simulink model "System"  (R2018b)
settings: Solver=FixedStepDiscrete  StartTime=0.0  StopTime=10  RelTol=1e-3
libraries: dspsrcs4 x3
settings Model: Creator=Whtest  LastModifiedBy=Whtest
settings OptimizationCC: DefaultParameterBehavior=Inlined  UseDivisionForNetSlopeComputation=on  UseFloatMulNetSlope=on  InlineInvariantSignals=on  PassReuseOutputArgsAs=Individual arguments  ZeroExternalMemoryAtStartup=off  ZeroInternalMemoryAtStartup=off  NoFixptDivByZeroProtection=on  EfficientFloat2IntCast=on  LifeSpan=1  OptimizeBlockOrder=speed  DifferentSizesBufferReuse=on
settings DebuggingCC: ParameterTunabilityLossMsg=error
settings HardwareCC: ProdBitPerPointer=32  ProdBitPerSizeT=32  ProdBitPerPtrDiffT=32  ProdWordSize=32  ProdLongLongMode=on  ProdHWDeviceType=Intel->x86-32 (Windows32)
settings SFSimCC: MATLABDynamicMemAlloc=off
settings RTWCC: SystemTargetFile=ert.tlc  TemplateMakefile=ert_default_tmf  GenerateReport=on  IncludeHyperlinkInReport=on  LaunchReport=on  GenerateTraceInfo=on  GenerateTraceReport=on  GenerateTraceReportSl=on  GenerateTraceReportSf=on  GenerateTraceReportEml=on  GenerateCodeMetricsReport=on
settings CodeAppCC: ForceParamTrailComments=on  IgnoreCustomStorageClasses=off  OperatorAnnotations=on  SimulinkDataObjDesc=on  SFDataObjDesc=on  CustomSymbolStrGlobalVar=rt$N$M  CustomSymbolStrType=$N$M  CustomSymbolStrFcn=$N$M$F  CustomSymbolStrMacro=$N$M  InsertBlockDesc=on
settings ERTTargetCC: TargetLangStandard=C99 (ISO)  GenerateSampleERTMain=on  IncludeMdlTerminateFcn=off  CombineSignalStateStructs=on  SupportComplex=off  SupportNonInlinedSFcns=on  InlinedParameterPlacement=NonHierarchical  ERTCustomFileTemplate=example_file_process.tlc  ERTFilePackagingFormat=CompactWithDataFile

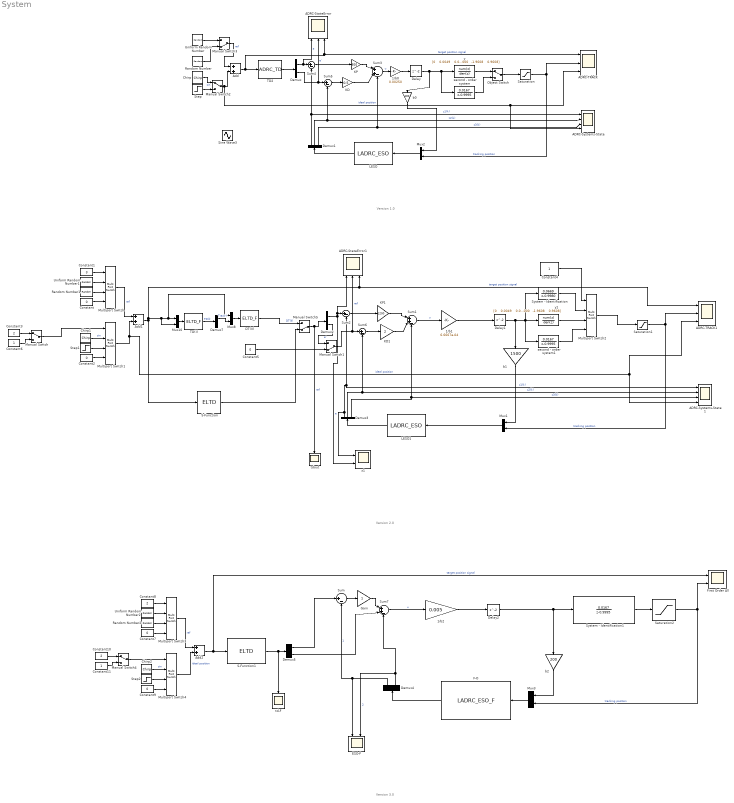
== system System ==
  note: Version 1.0
  note: Version 2.0
  note: Version 3.0
  1/b0 : Gain  Gain=0.00250
  1/b1 : Gain  Gain=6.6667e-04
  1/b2 : Gain  Gain=0.005
  ADRC-StateError : Scope  NumInputPorts=3
  ADRC-StateError1 : Scope  NumInputPorts=3
  "ADRC-Systems-State " : Scope  NumInputPorts=4
  ADRC-Systems-State 1 : Scope  NumInputPorts=4
  ADRC-TRACK : Scope  NumInputPorts=3
  ADRC-TRACK1 : Scope  NumInputPorts=3
  Add : Sum
  Add1 : Sum
  Add2 : Sum
  Chirp : dspsrcs4/Chirp  sweep=Linear  mode=Unidirectional  f0=1  f1=5  t1=5  Tsweep=5  phase=1.5*pi  Ts=0.001  spf=1  datatype=Double  OutputFrames=off
      settings: SourceProductName=DSP System Toolbox
  Chirp1 : dspsrcs4/Chirp  sweep=Linear  mode=Unidirectional  f0=1  f1=5  t1=5  Tsweep=5  phase=1.5*pi  Ts=0.001  spf=1  datatype=Double  OutputFrames=off
      settings: SourceProductName=DSP System Toolbox
  Chirp2 : dspsrcs4/Chirp  sweep=Linear  mode=Unidirectional  f0=1  f1=5  t1=5  Tsweep=5  phase=1.5*pi  Ts=0.001  spf=1  datatype=Double  OutputFrames=off
      settings: SourceProductName=DSP System Toolbox
  Constant{,2,5,7,9} (5 alike) : Constant  Value=0
  Constant1 : Constant  Value=3
  Constant10 : Constant  Value=2
  Constant11 : Constant
  Constant3 : Constant  Value=2
  Constant4 : Constant
  Constant6 : Constant
  Constant8 : Constant  Value=2
  DT(II) : S-Function  FunctionName=ELTD_F  Parameters=1,4,100,10  SFunctionDeploymentMode=off  EnableBusSupport=off
  Delay : Delay
  Delay1 : Delay
  Delay2 : Delay
  Demux{,2,4..5,7} (5 alike) : Demux  Outputs=2
  Demux1 : Demux  Outputs=3
  Demux3 : Demux  Outputs=3
  "ESO-F " : Scope  NumInputPorts=2
  F-O : S-Function  FunctionName=LADRC_ESO_F  Parameters=180,10800  SFunctionDeploymentMode=off  EnableBusSupport=off
  First Order All : Scope  NumInputPorts=2
  Gain : Gain
  KD : Gain  Gain=0.5
  KD1 : Gain  Gain=2
  KP : Gain  Gain=300
  KP1 : Gain  Gain=1200
  LESO : S-Function  FunctionName=LADRC_ESO  Parameters=100,300,1000  SFunctionDeploymentMode=off  EnableBusSupport=off
  LESO1 : S-Function  FunctionName=LADRC_ESO  Parameters=180,2160,24000  SFunctionDeploymentMode=off  EnableBusSupport=off
  Manual Switch : ManualSwitch
  Manual Switch1 : ManualSwitch  CurrentSetting=0
  Manual Switch2 : ManualSwitch
  Manual Switch3 : ManualSwitch  CurrentSetting=0
  Manual Switch4 : ManualSwitch
  Manual Switch5 : ManualSwitch  CurrentSetting=0
  Multiport Switch{,1..4} (5 alike) : MultiPortSwitch
  Mux{1..3,8,10} (5 alike) : Mux  Inputs=2
  Object Switch : ManualSwitch
  Random Number : RandomNumber  Variance=0.01  SampleTime=0.001
  Random Number1 : RandomNumber  Variance=0.01  SampleTime=0.001
  Random Number2 : RandomNumber  Variance=0.01  SampleTime=0.001
  S-Function : S-Function  FunctionName=ELTD  Parameters=1.2,4,100  SFunctionDeploymentMode=off  EnableBusSupport=off
  S-Function1 : S-Function  FunctionName=ELTD  Parameters=1.2,2,200  SFunctionDeploymentMode=off  EnableBusSupport=off
  Saturation : Saturate  UpperLimit=1000  LowerLimit=-1000
  Saturation1 : Saturate  UpperLimit=1e4  LowerLimit=-1e4
  Saturation2 : Saturate  UpperLimit=1e4  LowerLimit=-1e4
  Sine Wave3 : Sin  Frequency=3.14  SampleTime=1e-3
  Step : Step  After=10  SampleTime=1e-3
  Step1 : Step  After=2  SampleTime=5e-4
  Step2 : Step  After=2  SampleTime=5e-4
  Sum{,2,4..6} (5 alike) : Sum  Inputs=|+-
  Sum1 : Sum  Inputs=|++-
  Sum3 : Sum  Inputs=|++-
  Sum7 : Sum  Inputs=|++-
  System - Identification : DiscreteTransferFcn  Numerator="[0    0.0669]"  Denominator="[1.0000   -0.9980]"
  System - Identification1 : DiscreteTransferFcn  Numerator="[ 0    0.0167]"  Denominator="[1.0000   -0.9995]"
  TD(I) : S-Function  FunctionName=ELTD_F  Parameters=2.2,1.3,50,10  SFunctionDeploymentMode=off  EnableBusSupport=off
  TD2 : S-Function  FunctionName=ADRC_TD  Parameters=1e-2,5e6  SFunctionDeploymentMode=off  EnableBusSupport=off
  Uniform Random Number : UniformRandomNumber  Minimum=-0.1  Maximum=0.1  SampleTime=0.1
  Uniform Random Number1 : UniformRandomNumber  SampleTime=0.001
  Uniform Random Number2 : UniformRandomNumber  SampleTime=0.001
  b0 : Gain  Gain=400
  b1 : Gain  Gain=1500
  b2 : Gain  Gain=200
  second - order system : DiscreteTransferFcn  Numerator="[0    0.0167]"  Denominator="[1.0000   -0.9995]"
  second - order system1 : DiscreteTransferFcn  Numerator="[0    0.0167]"  Denominator="[1.0000   -0.9995]"
  "td-F " : Scope
  "tdout " : Scope
  "x1 " : Scope  NumInputPorts=2
  y : DiscreteTransferFcn  Numerator="[0    0.0049    0.0049]"  Denominator="[1.0000   -1.9608    0.9608]"
  y1 : DiscreteTransferFcn  Numerator="[0    0.0049    0.0049]"  Denominator="[1.0000   -1.9608    0.9608]"
  wires:
  Add/1 -> ADRC-StateError/3, ADRC-TRACK/1, TD2/1  "target position signal"
  TD2/1 -> Demux/1
  KP/1 -> Sum3/1
  KD/1 -> Sum3/2
  Sum3/1 -> 1/b0/1  "u"
  Sum4/1 -> KP/1
  Demux/2 -> Sum5/1, ADRC-StateError/2  "e'"
  Sum5/1 -> KD/1
  Demux1/3 -> Sum3/3, "ADRC-Systems-State "/3  "z3(k)"
  Demux1/2 -> Sum5/2, "ADRC-Systems-State "/2  "z2(k)"
  Demux1/1 -> "ADRC-Systems-State "/1, Sum4/2  "z1(k)"
  b0/1 -> Mux2/1
  Delay/1 -> b0/1, second - order system/1, y/1
  y/1 -> Object Switch/1
  second - order system/1 -> Object Switch/2
  Object Switch/1 -> Saturation/1
  Step/1 -> Manual Switch2/2
  Chirp/1 -> Manual Switch2/1  "sin"
  Manual Switch2/1 -> "ADRC-Systems-State "/4, ADRC-TRACK/3, Add/2  "ideal position"
  Random Number/1 -> Manual Switch3/2
  Mux2/1 -> LESO/1
  LESO/1 -> Demux1/1
  Saturation/1 -> Mux2/2, ADRC-TRACK/2  "tracking position"
  Demux/1 -> ADRC-StateError/1, Sum4/1  "e"
  1/b0/1 -> Delay/1
  Uniform Random Number/1 -> Manual Switch3/1
  Manual Switch3/1 -> Add/1  "ref"
  Chirp1/1 -> Multiport Switch1/2  "sin"
  1/b1/1 -> Delay1/1
  Demux2/1 -> ADRC-StateError1/1, Sum2/1, "x1 "/2  "e"
  LESO1/1 -> Demux3/1
  Mux1/1 -> LESO1/1
  Uniform Random Number1/1 -> Multiport Switch/2
  Add1/1 -> Mux10/2, Mux8/1, Mux10/1, ADRC-TRACK1/1, ADRC-StateError1/3, S-Function/1  "target position signal"
  Sum6/1 -> KD1/1
  b1/1 -> Mux1/1
  Demux3/1 -> ADRC-Systems-State 1/1, Sum2/2, "x1 "/1  "z1(k)"
  Demux3/2 -> ADRC-Systems-State 1/2, Sum6/2  "z2(k)"
  KP1/1 -> Sum1/1
  Demux3/3 -> Sum1/3, ADRC-Systems-State 1/3  "z3(k)"
  Sum1/1 -> 1/b1/1  "u"
  Sum2/1 -> KP1/1
  KD1/1 -> Sum1/2
  Multiport Switch1/1 -> ADRC-TRACK1/3, ADRC-Systems-State 1/4, Add1/2  "ideal position"
  Delay1/1 -> System - Identification/1, second - order system1/1, y1/1, b1/1
  S-Function/1 -> Manual Switch5/2
  Manual Switch5/1 -> "tdout "/1, Demux2/1  "ref"
  TD(I)/1 -> Demux7/1  "TD(I)"
  Mux10/1 -> TD(I)/1
  Demux7/1 -> Mux8/2  "Track-I"
  Mux8/1 -> DT(II)/1
  DT(II)/1 -> Manual Switch5/1  "DT(II)"
  Saturation1/1 -> Mux1/2, ADRC-TRACK1/2  "tracking position"
  second - order system1/1 -> Multiport Switch2/4
  y1/1 -> Multiport Switch2/3
  System - Identification/1 -> Multiport Switch2/2
  Multiport Switch/1 -> Add1/1  "ref"
  Random Number1/1 -> Multiport Switch/3
  Constant/1 -> Multiport Switch/4
  Constant1/1 -> Multiport Switch/1
  Step1/1 -> Multiport Switch1/3
  Constant2/1 -> Multiport Switch1/4
  Constant4/1 -> Multiport Switch2/1
  Multiport Switch2/1 -> Saturation1/1
  Demux2/2 -> Manual Switch1/1  "e'"
  Constant5/1 -> Manual Switch1/2
  Manual Switch1/1 -> ADRC-StateError1/2, Sum6/1  "ref"
  Constant3/1 -> Manual Switch/1
  Constant6/1 -> Manual Switch/2
  Manual Switch/1 -> Multiport Switch1/1
  Mux3/1 -> F-O/1
  1/b2/1 -> Delay2/1
  Delay2/1 -> System - Identification1/1, b2/1
  F-O/1 -> Demux4/1
  Multiport Switch3/1 -> Add2/1  "ref"
  Step2/1 -> Multiport Switch4/3
  Constant8/1 -> Multiport Switch3/1
  Constant7/1 -> Multiport Switch3/4
  Multiport Switch4/1 -> Add2/2  "ideal position"
  Random Number2/1 -> Multiport Switch3/3
  Uniform Random Number2/1 -> Multiport Switch3/2
  Manual Switch4/1 -> Multiport Switch4/1
  Constant10/1 -> Manual Switch4/1
  Constant9/1 -> Multiport Switch4/4
  Constant11/1 -> Manual Switch4/2
  Chirp2/1 -> Multiport Switch4/2  "sin"
  Add2/1 -> First Order All/1, S-Function1/1  "target position signal"
  S-Function1/1 -> "td-F "/1, Demux5/1
  System - Identification1/1 -> Saturation2/1
  Demux5/1 -> Sum/1
  Demux5/2 -> Sum7/2
  b2/1 -> Mux3/1
  Saturation2/1 -> Mux3/2, First Order All/2  "tracking position"
  Demux4/1 -> "ESO-F "/1, Sum/2  "1"
  Demux4/2 -> "ESO-F "/2, Sum7/3  "2"
  Sum7/1 -> 1/b2/1  "u"
  Sum/1 -> Gain/1
  Gain/1 -> Sum7/1
